simulink model "sl_pigle_Population"  (R2017b)
settings: Solver=FixedStepAuto  StartTime=0.0  StopTime=params.stop_time  FixedStep=params.sample_time  RelTol=1e-3  EnableMultiTasking=on
PreLoadFcn:
  | load pigle_data.mat
InitFcn:
  | load pigle_data.mat
undefined symbols (not defined in the file or in its folder): DiscIntNeverNeededParam, params
libraries: simulink x7, dspmtrx3 x2
settings Model: SnapshotBufferSize=1000  SnapshotInterval=1  OrderedModelArguments=off  Creator=na364  LastModifiedBy=na364
settings DataIOCC: LimitDataPoints=on
settings OptimizationCC: DefaultParameterBehavior=Inlined  LifeSpan=inf
settings DebuggingCC: AllowSymbolicDim=off  SFUnexpectedBacktrackingDiag=warning  SFNoUnconditionalDefaultTransitionDiag=warning  SFExecutionAtInitializationDiag=none
settings ModelReferenceCC: PropagateSignalLabelsOutOfModel=off
settings CodeAppCC: StateflowObjectComments=on
settings GRTTargetCC: TargetLangStandard=C89/C90 (ANSI)
settings ConfigComp: CovMetricSettings=dw  CovHtmlReporting=on  CovSaveCumulativeToWorkspaceVar=on  CovSaveSingleToWorkspaceVar=on  CovExternalEMLEnable=off
settings SimscapeCC: SimscapeNormalizeSystem=off
settings ConfigurationSet: Description=SimMechanics 2G

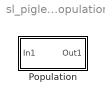
== system sl_pigle_Population ==
  Population : Subsystem

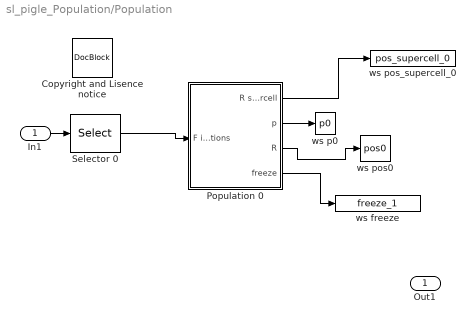
== system sl_pigle_Population/Population ==
  In1 : Inport
  Copyright and Lisence notice : simulink/Model-Wide Utilities/DocBlock  DocumentType=Text
      content=|
      | % Copyright (c) 2018, Nadav Avidor.
      | % All rights reserved.
      | % This file is part of the PIGLE - Particles Interacting in Generalized Langevin Equation simulator, subject to the
      | % GNU/GPL-3.0-or-later.
  Population 0 : Subsystem
  Selector 0 : Selector  NumberOfDimensions=2  InputPortWidth=3  IndexOptions=Select all,Starting index (dialog)  Indices=[1 3],1  OutputSizes=1,params.prtcl(1).Nprtcl
  ws freeze : ToWorkspace  VariableName=freeze_1  SampleTime=-1
      settings: Decimation=params.decimation
  ws p0 : ToWorkspace  VariableName=p0  SampleTime=-1
      settings: Decimation=params.decimation
  ws pos0 : ToWorkspace  VariableName=pos0  SampleTime=-1
      settings: Decimation=params.decimation
  ws pos_supercell_0 : ToWorkspace  VariableName=pos_supercell_0  SampleTime=-1
      settings: Decimation=params.decimation
  Out1 : Outport
  wires:
  Population 0/1(R supercell) -> ws pos_supercell_0/1
  Population 0/2(p) -> ws p0/1
  Population 0/3(R) -> ws pos0/1
  Selector 0/1 -> Population 0/1(F interactions)
  In1/1 -> Selector 0/1
  Population 0/4(freeze) -> ws freeze/1

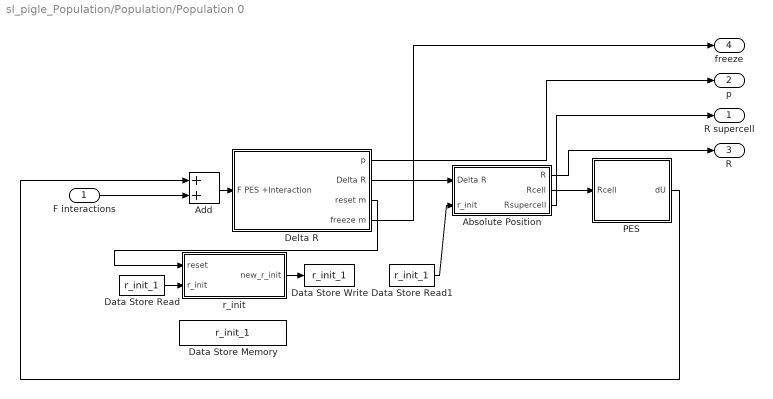
== system sl_pigle_Population/Population/Population 0 ==
  F interactions : Inport
  Absolute Position : Subsystem
  Add : Sum
  Data Store Memory : DataStoreMemory  DataStoreName=r_init_1  ReadBeforeWriteMsg=warning  WriteAfterWriteMsg=warning  WriteAfterReadMsg=warning  InitialValue=params.prtcl(1).r_init  VectorParams1D=off  ShowAdditionalParam=off
  Data Store Read : DataStoreRead  DataStoreName=r_init_1
  Data Store Read1 : DataStoreRead  DataStoreName=r_init_1
  Data Store Write : DataStoreWrite  DataStoreName=r_init_1
  Delta R : Subsystem
  PES : Subsystem
  r_init : Subsystem  TreatAsAtomicUnit=on
  R supercell : Outport
  p : Outport  Port=2
  R : Outport  Port=3
  freeze : Outport  Port=4
  wires:
  Add/1 -> Delta R/1(F PES +Interaction)
  F interactions/1 -> Add/2
  Absolute Position/1(R) -> R/1
  Absolute Position/3(Rsupercell) -> R supercell/1
  PES/1(dU) -> Add/1
  Delta R/1(p) -> p/1
  Delta R/2(Delta R) -> Absolute Position/1(Delta R)
  Absolute Position/2(Rcell) -> PES/1(Rcell)
  Delta R/3(reset m) -> r_init/1(reset)
  Data Store Read1/1 -> Absolute Position/2(r_init)
  Data Store Read/1 -> r_init/2(r_init)
  r_init/1(new_r_init) -> Data Store Write/1
  Delta R/4(freeze m) -> freeze/1

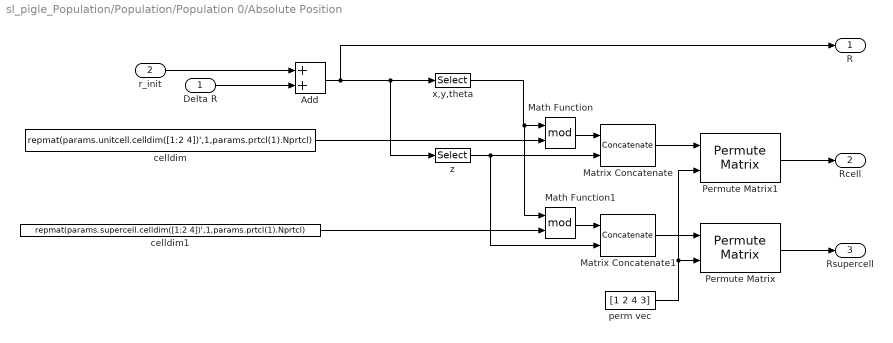
== system sl_pigle_Population/Population/Population 0/Absolute Position ==
  Delta R : Inport
  r_init : Inport  Port=2
  Add : Sum  Inputs=2
  Math Function : Math  Operator=mod  SaturateOnIntegerOverflow=on
  Math Function1 : Math  Operator=mod  SaturateOnIntegerOverflow=on
  Matrix Concatenate : Concatenate  Mode=Multidimensional array
  Matrix Concatenate1 : Concatenate  Mode=Multidimensional array
  Permute Matrix : dspmtrx3/Permute Matrix  mode=Rows  ZeroOneIdxMode=One-based  errmode=Generate error  checkDims=on
      settings: SourceProductName=DSP System Toolbox  SourceProductBaseCode=DS
  Permute Matrix1 : dspmtrx3/Permute Matrix  mode=Rows  ZeroOneIdxMode=One-based  errmode=Generate error  checkDims=on
      settings: SourceProductName=DSP System Toolbox  SourceProductBaseCode=DS
  celldim : Constant  Value=repmat(params.unitcell.celldim([1:2 4])',1,params.prtcl(1).Nprtcl)
  celldim1 : Constant  Value=repmat(params.supercell.celldim([1:2 4])',1,params.prtcl(1).Nprtcl)
  perm vec : Constant  Value=[1 2 4 3]
  x,y,theta : Selector  NumberOfDimensions=2  InputPortWidth=3  IndexOptions=Index vector (dialog),Select all  Indices=[1:2 4],1  OutputSizes=1,1
  z : Selector  NumberOfDimensions=2  InputPortWidth=3  IndexOptions=Index vector (dialog),Select all  Indices=3,1  OutputSizes=1,1
  R : Outport
  Rcell : Outport  Port=2
  Rsupercell : Outport  Port=3
  wires:
  celldim/1 -> Math Function/2
  r_init/1 -> Add/1
  Delta R/1 -> Add/2
  celldim1/1 -> Math Function1/2
  Add/1 -> z/1, x,y,theta/1, R/1
  Matrix Concatenate1/1 -> Permute Matrix/1
  Math Function1/1 -> Matrix Concatenate1/1
  x,y,theta/1 -> Math Function1/1, Math Function/1
  Math Function/1 -> Matrix Concatenate/1
  z/1 -> Matrix Concatenate1/2, Matrix Concatenate/2
  Permute Matrix/1 -> Rsupercell/1
  Permute Matrix1/1 -> Rcell/1
  perm vec/1 -> Permute Matrix/2, Permute Matrix1/2
  Matrix Concatenate/1 -> Permute Matrix1/1

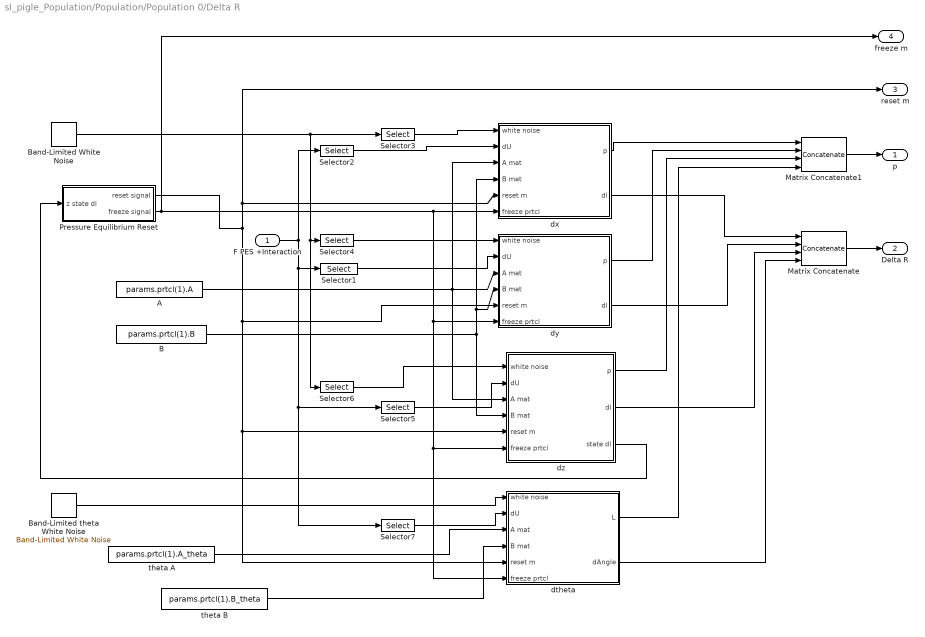
== system sl_pigle_Population/Population/Population 0/Delta R ==
  F PES +Interaction : Inport
  A : Constant  Value=params.prtcl(1).A  VectorParams1D=off
  B : Constant  Value=params.prtcl(1).B  VectorParams1D=off
  Band-Limited White Noise : simulink/Sources/Band-Limited White Noise  Cov=1  Ts=params.sample_time  seed=seed_values_1  VectorParams1D=off
  Band-Limited theta White Noise : simulink/Sources/Band-Limited White Noise  Cov=1  Ts=params.sample_time  seed=theta_seed_values_1  VectorParams1D=off
  Matrix Concatenate : Concatenate  NumInputs=4  Mode=Multidimensional array
  Matrix Concatenate1 : Concatenate  NumInputs=4  Mode=Multidimensional array
  Pressure Equilibrium Reset : Subsystem
  Selector1 : Selector  NumberOfDimensions=2  InputPortWidth=2  IndexOptions=Index vector (dialog),Select all  Indices=2,1  OutputSizes=1,1
  Selector2 : Selector  NumberOfDimensions=2  InputPortWidth=2  IndexOptions=Index vector (dialog),Select all  Indices=[1],1  OutputSizes=1,1
  Selector3 : Selector  NumberOfDimensions=3  InputPortWidth=2  IndexOptions=Select all,Select all,Index vector (dialog)  Indices=[1],1,1  OutputSizes=1,1,1
  Selector4 : Selector  NumberOfDimensions=3  InputPortWidth=2  IndexOptions=Select all,Select all,Index vector (dialog)  Indices=[1],1,2  OutputSizes=1,1,1
  Selector5 : Selector  NumberOfDimensions=2  InputPortWidth=2  IndexOptions=Index vector (dialog),Select all  Indices=3,1  OutputSizes=1,1
  Selector6 : Selector  NumberOfDimensions=3  InputPortWidth=2  IndexOptions=Select all,Select all,Index vector (dialog)  Indices=[1],1,3  OutputSizes=1,1,1
  Selector7 : Selector  NumberOfDimensions=2  InputPortWidth=2  IndexOptions=Index vector (dialog),Select all  Indices=4,1  OutputSizes=1,1
  dtheta : Subsystem
  dx : Subsystem
  dy : Subsystem
  dz : Subsystem
  theta A : Constant  Value=params.prtcl(1).A_theta  VectorParams1D=off
  theta B : Constant  Value=params.prtcl(1).B_theta  VectorParams1D=off
  p : Outport
  Delta R : Outport  Port=2
  reset m : Outport  Port=3
  freeze m : Outport  Port=4
  wires:
  A/1 -> dz/3(A mat), dx/3(A mat), dy/3(A mat)
  dx/1(p) -> Matrix Concatenate1/1
  dy/1(p) -> Matrix Concatenate1/2
  Band-Limited White Noise/1 -> Selector6/1, Selector4/1, Selector3/1
  Matrix Concatenate1/1 -> p/1
  Selector3/1 -> dx/1(white noise)
  dx/2(dl) -> Matrix Concatenate/1
  Matrix Concatenate/1 -> Delta R/1
  Selector2/1 -> dx/2(dU)
  Selector1/1 -> dy/2(dU)
  Selector4/1 -> dy/1(white noise)
  dy/2(dl) -> Matrix Concatenate/2
  F PES +Interaction/1 -> Selector2/1, Selector7/1, Selector5/1, Selector1/1
  B/1 -> dx/4(B mat), dy/4(B mat), dz/4(B mat)
  Selector6/1 -> dz/1(white noise)
  Selector5/1 -> dz/2(dU)
  Selector7/1 -> dtheta/2(dU)
  theta B/1 -> dtheta/4(B mat)
  theta A/1 -> dtheta/3(A mat)
  Band-Limited theta White Noise/1 -> dtheta/1(white noise)
  dtheta/2(dAngle) -> Matrix Concatenate/4
  dtheta/1(L) -> Matrix Concatenate1/4
  dz/2(dl) -> Matrix Concatenate/3
  dz/1(p) -> Matrix Concatenate1/3
  Pressure Equilibrium Reset/1(reset signal) -> dy/5(reset m), dz/5(reset m), dtheta/5(reset m), reset m/1, dx/5(reset m)
  dz/3(state dl) -> Pressure Equilibrium Reset/1(z state dl)
  Pressure Equilibrium Reset/2(freeze signal) -> dy/6(freeze prtcl), dtheta/6(freeze prtcl), dz/6(freeze prtcl), dx/6(freeze prtcl), freeze m/1

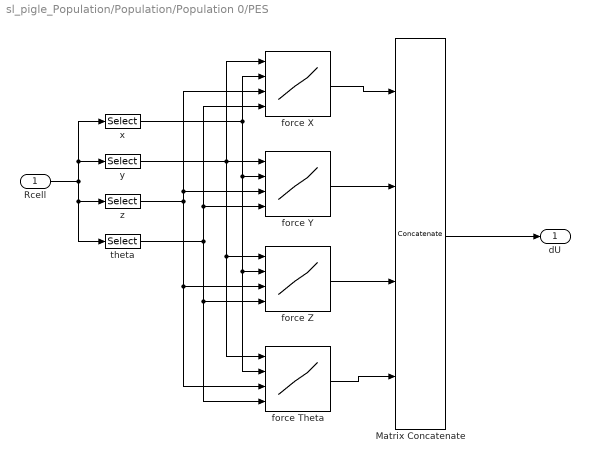
== system sl_pigle_Population/Population/Population 0/PES ==
  Rcell : Inport
  Matrix Concatenate : Concatenate  NumInputs=4  Mode=Multidimensional array
  force Theta : Lookup_n-D  NumberOfTableDimensions=4  BreakpointsForDimension1=params.unitcell.y  BreakpointsForDimension2=params.unitcell.x  BreakpointsForDimension3=params.unitcell.z  BreakpointsForDimension4=params.unitcell.theta  Table=params.prtcl(1).pes.ftheta  InternalRulePriority=Speed  RndMeth=Simplest  InputSameDT=on
  force X : Lookup_n-D  NumberOfTableDimensions=4  BreakpointsForDimension1=params.unitcell.y  BreakpointsForDimension2=params.unitcell.x  BreakpointsForDimension3=params.unitcell.z  BreakpointsForDimension4=params.unitcell.theta  Table=params.prtcl(1).pes.fx  InternalRulePriority=Speed  RndMeth=Simplest  InputSameDT=on
  force Y : Lookup_n-D  NumberOfTableDimensions=4  BreakpointsForDimension1=params.unitcell.y  BreakpointsForDimension2=params.unitcell.x  BreakpointsForDimension3=params.unitcell.z  BreakpointsForDimension4=params.unitcell.theta  Table=params.prtcl(1).pes.fy  InternalRulePriority=Speed  RndMeth=Simplest  InputSameDT=on
  force Z : Lookup_n-D  NumberOfTableDimensions=4  BreakpointsForDimension1=params.unitcell.y  BreakpointsForDimension2=params.unitcell.x  BreakpointsForDimension3=params.unitcell.z  BreakpointsForDimension4=params.unitcell.theta  Table=params.prtcl(1).pes.fz  InternalRulePriority=Speed  RndMeth=Simplest  InputSameDT=on
  theta : Selector  NumberOfDimensions=2  InputPortWidth=3  IndexOptions=Index vector (dialog),Select all  Indices=4,1  OutputSizes=1,1
  x : Selector  NumberOfDimensions=2  InputPortWidth=3  IndexOptions=Index vector (dialog),Select all  Indices=1,1  OutputSizes=1,1
  y : Selector  NumberOfDimensions=2  InputPortWidth=3  IndexOptions=Index vector (dialog),Select all  Indices=2,1  OutputSizes=1,1
  z : Selector  NumberOfDimensions=2  InputPortWidth=3  IndexOptions=Index vector (dialog),Select all  Indices=3,1  OutputSizes=1,1
  dU : Outport
  wires:
  force X/1 -> Matrix Concatenate/1
  y/1 -> force Theta/1, force Z/1, force Y/1, force X/1
  force Y/1 -> Matrix Concatenate/2
  x/1 -> force Theta/2, force Z/2, force Y/2, force X/2
  Rcell/1 -> x/1, y/1, theta/1, z/1
  Matrix Concatenate/1 -> dU/1
  z/1 -> force Z/3, force Theta/3, force Y/3, force X/3
  theta/1 -> force Y/4, force X/4, force Theta/4, force Z/4
  force Theta/1 -> Matrix Concatenate/4
  force Z/1 -> Matrix Concatenate/3

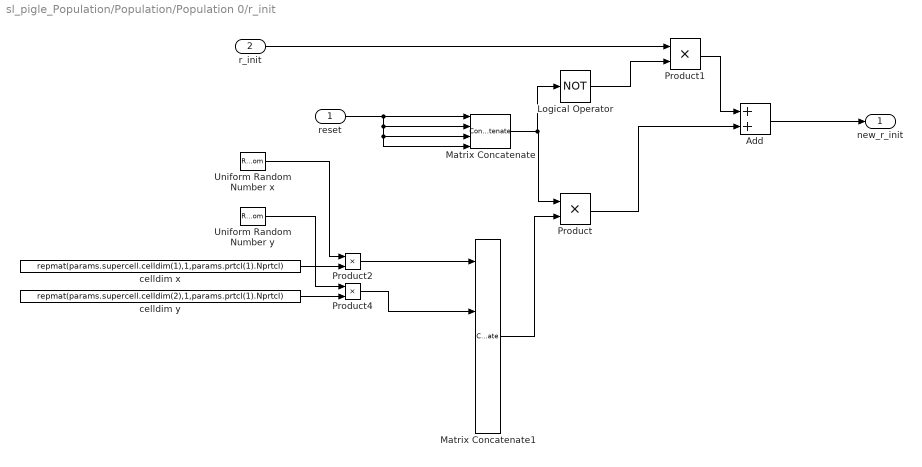
== system sl_pigle_Population/Population/Population 0/r_init ==
  reset : Inport
  r_init : Inport  Port=2
  Add : Sum
  Logical Operator : Logic  Operator=NOT  AllPortsSameDT=off  OutDataTypeStr=boolean
  Matrix Concatenate : Concatenate  NumInputs=4  Mode=Multidimensional array
  Matrix Concatenate1 : Concatenate  NumInputs=4  Mode=Multidimensional array
  Product{,1..2,4} (4 alike) : Product
  Uniform Random Number x : UniformRandomNumber  Minimum=0  Seed=randi(100000,1,params.prtcl(1).Nprtcl)  SampleTime=params.sample_time
  Uniform Random Number y : UniformRandomNumber  Minimum=0  Seed=randi(100000,1,params.prtcl(1).Nprtcl)  SampleTime=params.sample_time
  celldim x : Constant  Value=repmat(params.supercell.celldim(1),1,params.prtcl(1).Nprtcl)  VectorParams1D=off
  celldim y : Constant  Value=repmat(params.supercell.celldim(2),1,params.prtcl(1).Nprtcl)  VectorParams1D=off
  new_r_init : Outport
  wires:
  Matrix Concatenate/1 -> Logical Operator/1, Product/1
  Add/1 -> new_r_init/1
  Matrix Concatenate1/1 -> Product/2
  Product/1 -> Add/2
  reset/1 -> Matrix Concatenate/3, Matrix Concatenate/4, Matrix Concatenate/2, Matrix Concatenate/1
  Product1/1 -> Add/1
  Logical Operator/1 -> Product1/2
  celldim x/1 -> Product2/2
  Product2/1 -> Matrix Concatenate1/1
  Uniform Random Number x/1 -> Product2/1
  Product4/1 -> Matrix Concatenate1/2
  r_init/1 -> Product1/1
  Uniform Random Number y/1 -> Product4/1
  celldim y/1 -> Product4/2

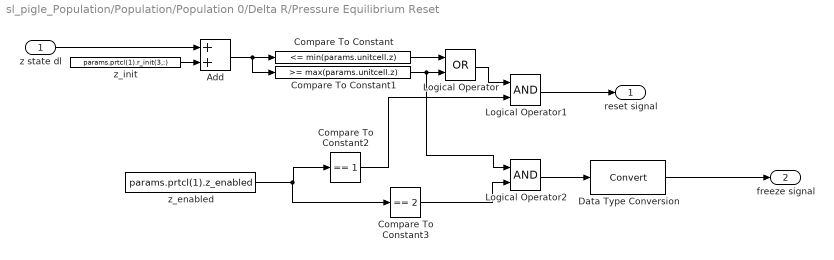
== system sl_pigle_Population/Population/Population 0/Delta R/Pressure Equilibrium Reset ==
  z state dl : Inport
  Add : Sum  Inputs=2
  Compare To Constant : simulink/Logic and Bit Operations/Compare To Constant  relop=<=  const=min(params.unitcell.z)  OutDataTypeStr=boolean
  Compare To Constant1 : simulink/Logic and Bit Operations/Compare To Constant  relop=>=  const=max(params.unitcell.z)  OutDataTypeStr=boolean
  Compare To Constant2 : simulink/Logic and Bit Operations/Compare To Constant  relop===  const=1  OutDataTypeStr=boolean
  Compare To Constant3 : simulink/Logic and Bit Operations/Compare To Constant  relop===  const=2  OutDataTypeStr=boolean
  Data Type Conversion : DataTypeConversion
  Logical Operator : Logic  Operator=OR  AllPortsSameDT=off  OutDataTypeStr=fixdt(1,16)
  Logical Operator1 : Logic  AllPortsSameDT=off  OutDataTypeStr=fixdt(1,16)
  Logical Operator2 : Logic  AllPortsSameDT=off  OutDataTypeStr=fixdt(1,16)
  z_enabled : Constant  Value=params.prtcl(1).z_enabled  VectorParams1D=off
  z_init : Constant  Value=params.prtcl(1).r_init(3,:)  VectorParams1D=off
  reset signal : Outport
  freeze signal : Outport  Port=2
  wires:
  Logical Operator/1 -> Logical Operator1/1
  Compare To Constant/1 -> Logical Operator/1
  z_enabled/1 -> Compare To Constant3/1, Compare To Constant2/1
  z_init/1 -> Add/2
  Compare To Constant1/1 -> Logical Operator2/1, Logical Operator/2
  z state dl/1 -> Add/1
  Add/1 -> Compare To Constant1/1, Compare To Constant/1
  Logical Operator1/1 -> reset signal/1
  Compare To Constant2/1 -> Logical Operator1/2
  Compare To Constant3/1 -> Logical Operator2/2
  Logical Operator2/1 -> Data Type Conversion/1
  Data Type Conversion/1 -> freeze signal/1

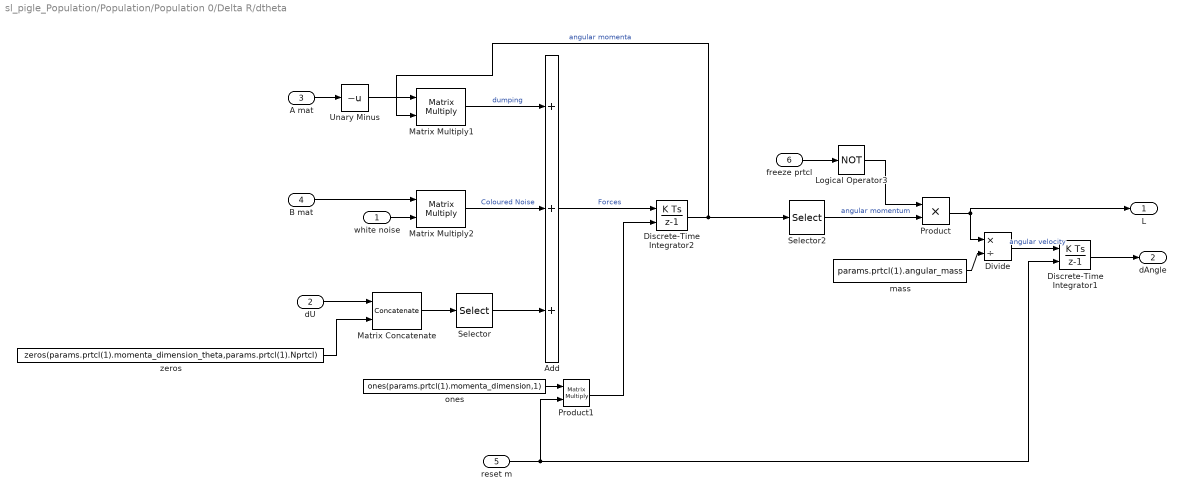
== system sl_pigle_Population/Population/Population 0/Delta R/dtheta ==
  white noise : Inport
  dU : Inport  Port=2
  A mat : Inport  Port=3
  B mat : Inport  Port=4
  reset m : Inport  Port=5
  freeze prtcl : Inport  Port=6
  Add : Sum  Inputs=+++
  Discrete-Time Integrator1 : DiscreteIntegrator  ExternalReset=sampled level  InitialConditionSetting=State (most efficient)  SampleTime=-1  ICPrevOutput=DiscIntNeverNeededParam  ICPrevScaledInput=DiscIntNeverNeededParam
  Discrete-Time Integrator2 : DiscreteIntegrator  ExternalReset=sampled level  InitialConditionSetting=State (most efficient)  SampleTime=-1  ICPrevOutput=DiscIntNeverNeededParam  ICPrevScaledInput=DiscIntNeverNeededParam
  Divide : Product  Inputs=*/
  Logical Operator3 : Logic  Operator=NOT  AllPortsSameDT=off  OutDataTypeStr=fixdt(1,16)
  Matrix Concatenate : Concatenate  Mode=Multidimensional array
  Matrix Multiply1 : Product  Multiplication=Matrix(*)
  Matrix Multiply2 : Product  Multiplication=Matrix(*)
  Product : Product
  Product1 : Product  Multiplication=Matrix(*)
  Selector : Selector  NumberOfDimensions=2  InputPortWidth=2  IndexOptions=Index vector (dialog),Index vector (dialog)  Indices=1:params.prtcl(1).momenta_dimension_theta,1:params.prtcl(1).Nprtcl  OutputSizes=1,1
  Selector2 : Selector  NumberOfDimensions=2  InputPortWidth=2  IndexOptions=Index vector (dialog),Select all  Indices=1,1  OutputSizes=1,1
  Unary Minus : UnaryMinus
  mass : Constant  Value=params.prtcl(1).angular_mass
  ones : Constant  Value=ones(params.prtcl(1).momenta_dimension,1)  VectorParams1D=off
  zeros : Constant  Value=zeros(params.prtcl(1).momenta_dimension_theta,params.prtcl(1).Nprtcl)  VectorParams1D=off
  L : Outport
  dAngle : Outport  Port=2
  wires:
  zeros/1 -> Matrix Concatenate/2
  Unary Minus/1 -> Matrix Multiply1/1
  Divide/1 -> Discrete-Time Integrator1/1  "angular velocity"
  mass/1 -> Divide/2
  Matrix Concatenate/1 -> Selector/1
  Discrete-Time Integrator2/1 -> Selector2/1, Matrix Multiply1/2  "angular momenta"
  Selector/1 -> Add/3
  white noise/1 -> Matrix Multiply2/2
  A mat/1 -> Unary Minus/1
  B mat/1 -> Matrix Multiply2/1
  Add/1 -> Discrete-Time Integrator2/1  "Forces"
  Product/1 -> L/1, Divide/1
  Matrix Multiply1/1 -> Add/1  "dumping"
  Discrete-Time Integrator1/1 -> dAngle/1
  Matrix Multiply2/1 -> Add/2  "Coloured Noise"
  dU/1 -> Matrix Concatenate/1
  reset m/1 -> Discrete-Time Integrator1/2, Product1/2
  freeze prtcl/1 -> Logical Operator3/1
  Selector2/1 -> Product/2  "angular momentum"
  ones/1 -> Product1/1
  Product1/1 -> Discrete-Time Integrator2/2
  Logical Operator3/1 -> Product/1

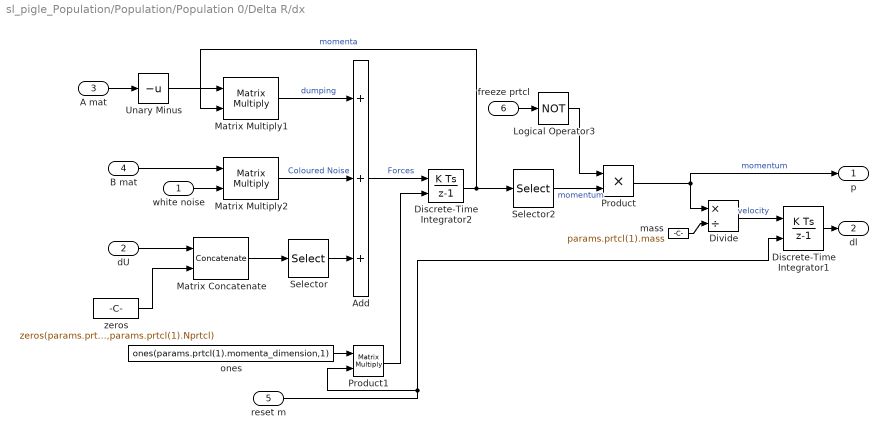
== system sl_pigle_Population/Population/Population 0/Delta R/dx ==
  white noise : Inport
  dU : Inport  Port=2
  A mat : Inport  Port=3
  B mat : Inport  Port=4
  reset m : Inport  Port=5
  freeze prtcl : Inport  Port=6
  Add : Sum  Inputs=+++
  Discrete-Time Integrator1 : DiscreteIntegrator  ExternalReset=sampled level  InitialConditionSetting=State (most efficient)  SampleTime=-1  ICPrevOutput=DiscIntNeverNeededParam  ICPrevScaledInput=DiscIntNeverNeededParam
  Discrete-Time Integrator2 : DiscreteIntegrator  ExternalReset=sampled level  InitialConditionSetting=State (most efficient)  SampleTime=-1  ICPrevOutput=DiscIntNeverNeededParam  ICPrevScaledInput=DiscIntNeverNeededParam
  Divide : Product  Inputs=*/
  Logical Operator3 : Logic  Operator=NOT  AllPortsSameDT=off  OutDataTypeStr=fixdt(1,16)
  Matrix Concatenate : Concatenate  Mode=Multidimensional array
  Matrix Multiply1 : Product  Multiplication=Matrix(*)
  Matrix Multiply2 : Product  Multiplication=Matrix(*)
  Product : Product
  Product1 : Product  Multiplication=Matrix(*)
  Selector : Selector  NumberOfDimensions=2  InputPortWidth=2  IndexOptions=Index vector (dialog),Index vector (dialog)  Indices=1:params.prtcl(1).momenta_dimension,1:params.prtcl(1).Nprtcl  OutputSizes=1,1
  Selector2 : Selector  NumberOfDimensions=2  InputPortWidth=2  IndexOptions=Index vector (dialog),Select all  Indices=1,1  OutputSizes=1,1
  Unary Minus : UnaryMinus
  mass : Constant  Value=params.prtcl(1).mass
  ones : Constant  Value=ones(params.prtcl(1).momenta_dimension,1)  VectorParams1D=off
  zeros : Constant  Value=zeros(params.prtcl(1).momenta_dimension,params.prtcl(1).Nprtcl)  VectorParams1D=off
  p : Outport
  dl : Outport  Port=2
  wires:
  zeros/1 -> Matrix Concatenate/2
  Unary Minus/1 -> Matrix Multiply1/1
  Divide/1 -> Discrete-Time Integrator1/1  "velocity"
  mass/1 -> Divide/2
  Matrix Concatenate/1 -> Selector/1
  Selector/1 -> Add/3
  white noise/1 -> Matrix Multiply2/2
  A mat/1 -> Unary Minus/1
  B mat/1 -> Matrix Multiply2/1
  Add/1 -> Discrete-Time Integrator2/1  "Forces"
  Product/1 -> p/1, Divide/1  "momentum"
  Matrix Multiply1/1 -> Add/1  "dumping"
  Discrete-Time Integrator1/1 -> dl/1
  Matrix Multiply2/1 -> Add/2  "Coloured Noise"
  dU/1 -> Matrix Concatenate/1
  reset m/1 -> Discrete-Time Integrator1/2, Product1/2
  freeze prtcl/1 -> Logical Operator3/1
  Discrete-Time Integrator2/1 -> Selector2/1, Matrix Multiply1/2  "momenta"
  Selector2/1 -> Product/2  "momentum"
  ones/1 -> Product1/1
  Product1/1 -> Discrete-Time Integrator2/2
  Logical Operator3/1 -> Product/1

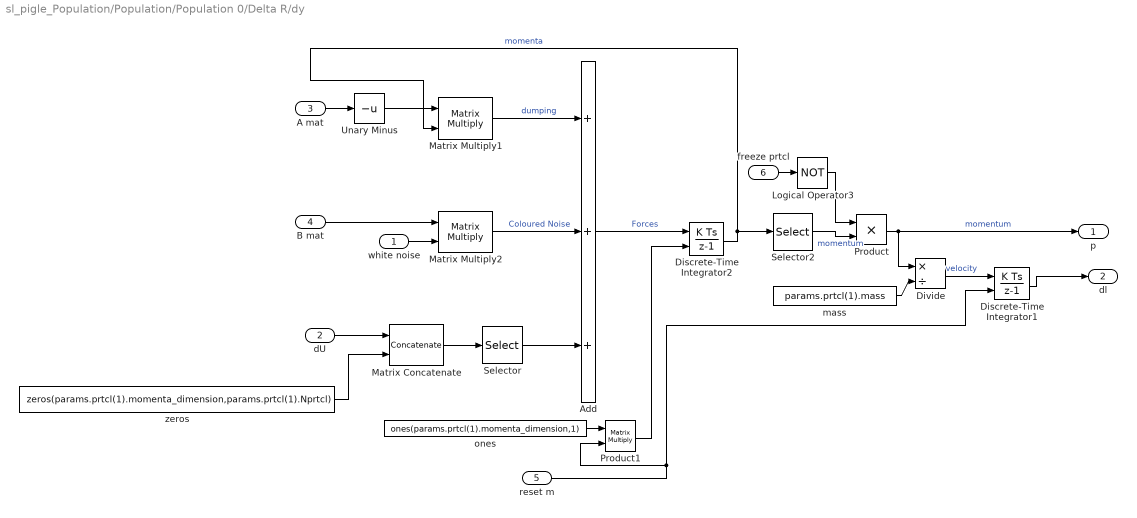
== system sl_pigle_Population/Population/Population 0/Delta R/dy ==
  white noise : Inport
  dU : Inport  Port=2
  A mat : Inport  Port=3
  B mat : Inport  Port=4
  reset m : Inport  Port=5
  freeze prtcl : Inport  Port=6
  Add : Sum  Inputs=+++
  Discrete-Time Integrator1 : DiscreteIntegrator  ExternalReset=sampled level  InitialConditionSetting=State (most efficient)  SampleTime=-1  ICPrevOutput=DiscIntNeverNeededParam  ICPrevScaledInput=DiscIntNeverNeededParam
  Discrete-Time Integrator2 : DiscreteIntegrator  ExternalReset=sampled level  InitialConditionSetting=State (most efficient)  SampleTime=-1  ICPrevOutput=DiscIntNeverNeededParam  ICPrevScaledInput=DiscIntNeverNeededParam
  Divide : Product  Inputs=*/
  Logical Operator3 : Logic  Operator=NOT  AllPortsSameDT=off  OutDataTypeStr=fixdt(1,16)
  Matrix Concatenate : Concatenate  Mode=Multidimensional array
  Matrix Multiply1 : Product  Multiplication=Matrix(*)
  Matrix Multiply2 : Product  Multiplication=Matrix(*)
  Product : Product
  Product1 : Product  Multiplication=Matrix(*)
  Selector : Selector  NumberOfDimensions=2  InputPortWidth=2  IndexOptions=Index vector (dialog),Index vector (dialog)  Indices=1:params.prtcl(1).momenta_dimension,1:params.prtcl(1).Nprtcl  OutputSizes=1,1
  Selector2 : Selector  NumberOfDimensions=2  InputPortWidth=2  IndexOptions=Index vector (dialog),Select all  Indices=1,1  OutputSizes=1,1
  Unary Minus : UnaryMinus
  mass : Constant  Value=params.prtcl(1).mass
  ones : Constant  Value=ones(params.prtcl(1).momenta_dimension,1)  VectorParams1D=off
  zeros : Constant  Value=zeros(params.prtcl(1).momenta_dimension,params.prtcl(1).Nprtcl)  VectorParams1D=off
  p : Outport
  dl : Outport  Port=2
  wires:
  zeros/1 -> Matrix Concatenate/2
  Unary Minus/1 -> Matrix Multiply1/1
  Divide/1 -> Discrete-Time Integrator1/1  "velocity"
  mass/1 -> Divide/2
  Matrix Concatenate/1 -> Selector/1
  Discrete-Time Integrator2/1 -> Matrix Multiply1/2, Selector2/1  "momenta"
  Selector/1 -> Add/3
  white noise/1 -> Matrix Multiply2/2
  A mat/1 -> Unary Minus/1
  B mat/1 -> Matrix Multiply2/1
  Add/1 -> Discrete-Time Integrator2/1  "Forces"
  Product/1 -> Divide/1, p/1  "momentum"
  Matrix Multiply1/1 -> Add/1  "dumping"
  Discrete-Time Integrator1/1 -> dl/1
  Matrix Multiply2/1 -> Add/2  "Coloured Noise"
  dU/1 -> Matrix Concatenate/1
  reset m/1 -> Discrete-Time Integrator1/2, Product1/2
  freeze prtcl/1 -> Logical Operator3/1
  Selector2/1 -> Product/2  "momentum"
  ones/1 -> Product1/1
  Product1/1 -> Discrete-Time Integrator2/2
  Logical Operator3/1 -> Product/1

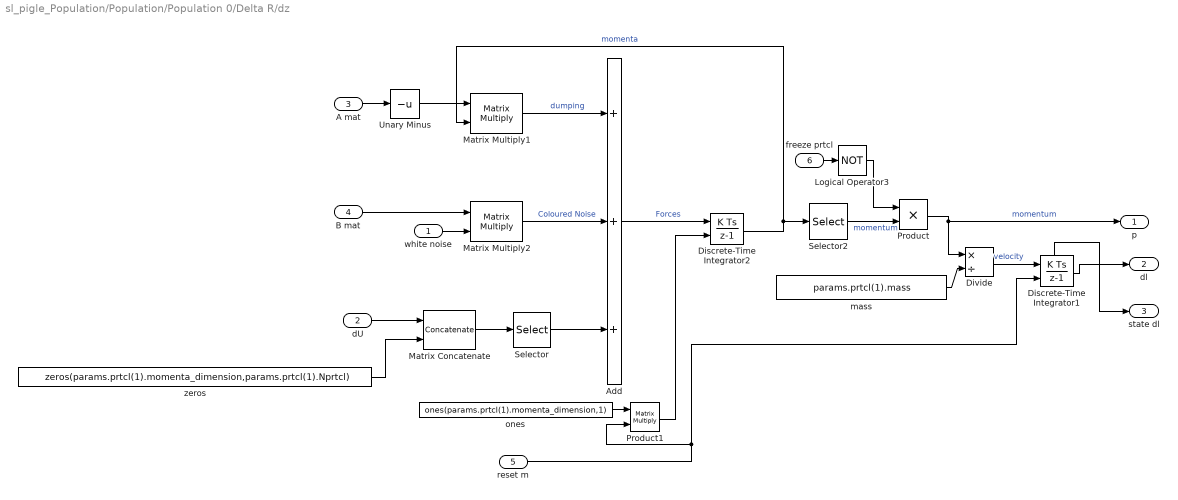
== system sl_pigle_Population/Population/Population 0/Delta R/dz ==
  white noise : Inport
  dU : Inport  Port=2
  A mat : Inport  Port=3
  B mat : Inport  Port=4
  reset m : Inport  Port=5
  freeze prtcl : Inport  Port=6
  Add : Sum  Inputs=+++
  Discrete-Time Integrator1 : DiscreteIntegrator  ExternalReset=level  InitialConditionSetting=State (most efficient)  SampleTime=-1  ShowStatePort=on  ICPrevOutput=DiscIntNeverNeededParam  ICPrevScaledInput=DiscIntNeverNeededParam
  Discrete-Time Integrator2 : DiscreteIntegrator  ExternalReset=level  InitialConditionSetting=State (most efficient)  SampleTime=-1  ICPrevOutput=DiscIntNeverNeededParam  ICPrevScaledInput=DiscIntNeverNeededParam
  Divide : Product  Inputs=*/
  Logical Operator3 : Logic  Operator=NOT  AllPortsSameDT=off  OutDataTypeStr=fixdt(1,16)
  Matrix Concatenate : Concatenate  Mode=Multidimensional array
  Matrix Multiply1 : Product  Multiplication=Matrix(*)
  Matrix Multiply2 : Product  Multiplication=Matrix(*)
  Product : Product
  Product1 : Product  Multiplication=Matrix(*)
  Selector : Selector  NumberOfDimensions=2  InputPortWidth=2  IndexOptions=Index vector (dialog),Index vector (dialog)  Indices=1:params.prtcl(1).momenta_dimension,1:params.prtcl(1).Nprtcl  OutputSizes=1,1
  Selector2 : Selector  NumberOfDimensions=2  InputPortWidth=2  IndexOptions=Index vector (dialog),Select all  Indices=1,1  OutputSizes=1,1
  Unary Minus : UnaryMinus
  mass : Constant  Value=params.prtcl(1).mass
  ones : Constant  Value=ones(params.prtcl(1).momenta_dimension,1)  VectorParams1D=off
  zeros : Constant  Value=zeros(params.prtcl(1).momenta_dimension,params.prtcl(1).Nprtcl)  VectorParams1D=off
  p : Outport
  dl : Outport  Port=2
  state dl : Outport  Port=3
  wires:
  zeros/1 -> Matrix Concatenate/2
  Unary Minus/1 -> Matrix Multiply1/1
  Divide/1 -> Discrete-Time Integrator1/1  "velocity"
  mass/1 -> Divide/2
  Matrix Concatenate/1 -> Selector/1
  Selector/1 -> Add/3
  white noise/1 -> Matrix Multiply2/2
  A mat/1 -> Unary Minus/1
  B mat/1 -> Matrix Multiply2/1
  Add/1 -> Discrete-Time Integrator2/1  "Forces"
  Product/1 -> p/1, Divide/1  "momentum"
  Matrix Multiply1/1 -> Add/1  "dumping"
  Discrete-Time Integrator1/1 -> dl/1
  Matrix Multiply2/1 -> Add/2  "Coloured Noise"
  dU/1 -> Matrix Concatenate/1
  Discrete-Time Integrator1/State -> state dl/1
  reset m/1 -> Discrete-Time Integrator1/2, Product1/2
  Logical Operator3/1 -> Product/1
  Discrete-Time Integrator2/1 -> Matrix Multiply1/2, Selector2/1  "momenta"
  Selector2/1 -> Product/2  "momentum"
  ones/1 -> Product1/1
  Product1/1 -> Discrete-Time Integrator2/2
  freeze prtcl/1 -> Logical Operator3/1
